simulink model "SimplifiedTF"  (R2017a)
settings: Solver=VariableStepAuto  StartTime=0.0  StopTime=10.0  RelTol=1e-3
undefined symbols (not defined in the file or in its folder): JmLa, JMLa, JmRa, JMRa, Kt, KtKe, Laf, Raf
settings Model: Creator=ni_daly  LastModifiedBy=ni_daly

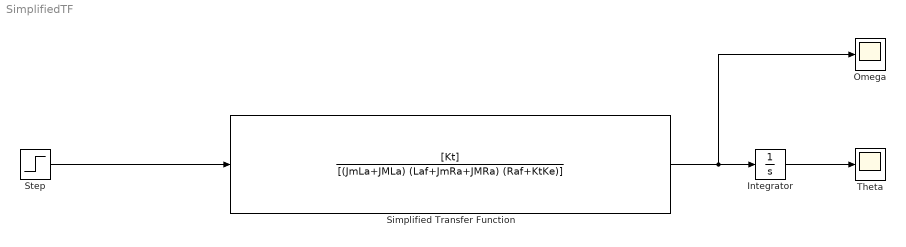
== system SimplifiedTF ==
  Integrator : Integrator
  Omega : Scope
  Simplified Transfer Function : TransferFcn  Numerator=[Kt]  Denominator=[(JmLa+JMLa) (Laf+JmRa+JMRa) (Raf+KtKe)]
  Step : Step  SampleTime=0
  Theta : Scope
  wires:
  Simplified Transfer Function/1 -> Integrator/1, Omega/1
  Integrator/1 -> Theta/1
  Step/1 -> Simplified Transfer Function/1
